simulink model "S"  (R2018b)
settings: Solver=ode14x  StartTime=0.0  StopTime=100  FixedStep=0.01  RelTol=1e-3
StopFcn:
  | figure;
  | plot(t,ref,'r--','linewidth',1.5);
  | hold on
  | plot(t,Ph,'k','linewidth',1.5);
  | legend('ref','Ph');
  | xlabel('events');ylabel('Ph(Mpa)');
  | grid on;
  | %%
  | figure
  | subplot(311)
  | plot(t,u,'k','linewidth',1);
  | ylabel('Voltage(v)');
  | hold on
  | legend('u')
  | grid on;
  | subplot(312)
  | plot(t,u_fbk,'k','linewidth',1.5);
  | ylabel('Voltage(v)');
  | legend('u_fbk');
  | hold on
  | grid on;
  | subplot(313)
  | plot(t,u_ffrk,'k','linewidth',1.5);
  | legend('u_ffrk');
  | xlabel('events');ylabel('Voltage(v)');
  | grid on;
  | %%
  | figure;
  | plot(t,rise,'k','linewidth',1.5);
  | hold on
  | plot(t,rise_r,'r--','linewidth',1.5);
  | legend('ref','Rising Duration');
  | xlabel('events');ylabel('Rising Duration(ms)');
  | grid on;
undefined symbols (not defined in the file or in its folder): sigbuilder_block
settings Model: Creator=sos h  LastModifiedBy=sistana
settings SolverCC: AlgebraicLoopSolver=LineSearch
settings SFSimCC: SimUseLocalCustomCode=off
settings RTWCC: RTWUseLocalCustomCode=off

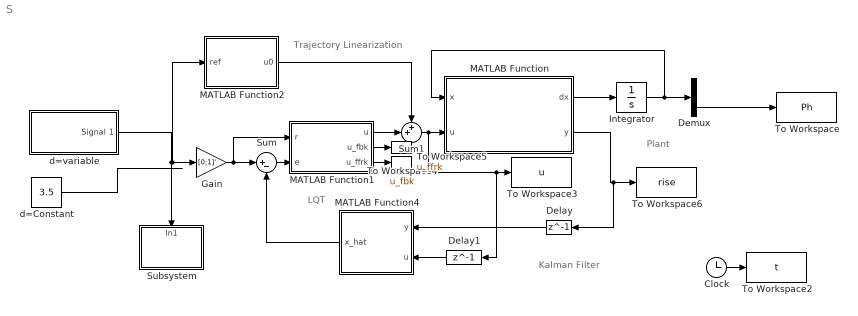
== system S ==
  note: Trajectory Linearization
  note: LQT
  note: Kalman Filter
  note: Plant
  Clock : Clock
  Delay : Delay  DelayLength=1
  Delay1 : Delay  DelayLength=1
  Demux : Demux  Outputs=2
  Gain : Gain  Gain=[0;1]'
  Integrator : Integrator  InitialCondition=[0.1;5]
  MATLAB Function : MATLAB Function  TreatAsAtomicUnit=on
  MATLAB Function1 : MATLAB Function  TreatAsAtomicUnit=on
  MATLAB Function2 : MATLAB Function  TreatAsAtomicUnit=on
  MATLAB Function4 : MATLAB Function  TreatAsAtomicUnit=on
  Subsystem : Subsystem
  Sum : Sum  Inputs=|+-
  Sum1 : Sum  Inputs=++|
  To Workspace : ToWorkspace  VariableName=Ph  SampleTime=-1
  To Workspace2 : ToWorkspace  VariableName=t  SampleTime=-1
  To Workspace3 : ToWorkspace  VariableName=u  SampleTime=-1
  To Workspace4 : ToWorkspace  VariableName=u_fbk  SampleTime=-1
  To Workspace5 : ToWorkspace  VariableName=u_ffrk  SampleTime=-1
  To Workspace6 : ToWorkspace  VariableName=rise  SampleTime=-1
  d=Constant : Constant  Value=3.5
  d=variable : Subsystem  Tag=STV Subsys  LoadFcn=sigbuilder_block('load');  StartFcn=sigbuilder_block('start');  StopFcn=sigbuilder_block('stop');  ClipboardFcn=sigbuilder_block('clipboard');  mask(Sigbuilder block){tuvar=[0:10]}
      mask help: Simulink:masks:SigbuilderBlock_MD
      mask init:
      | if ~strcmp(get_param(bdroot(gcbh),'SimulationStatus'),'stopped') tuvar = sigbuilder_block('maskInit'); end
      settings: CopyFcn=sigbuilder_block('copy');  DeleteFcn=sigbuilder_block('delete');  ModelCloseFcn=sigbuilder_block('modelClose');  PreSaveFcn=sigbuilder_block('preSave');  PauseFcn=sigbuilder_block('pause');  ContinueFcn=sigbuilder_block('continue');  NameChangeFcn=sigbuilder_block('namechange');  OpenFcn=sigbuilder_block('open',[437.25 153.75 550.5 359.25 ]);  CloseFcn=sigbuilder_block('close');
      mask Display: plot(0, 0, 100, 100,[2, 2, 32, 32, 2], [68, 8, 8, 68, 68],[32, 2], [38, 38], [32, 19, 2],[53, 60, 44], [32, 17, 17, 2],[16, 16, 31, 31]);txt = getActiveGroup(gcbh);text(2, 100, txt,'verticalAlignment', 'top');
  wires:
  MATLAB Function1/2(u_fbk) -> To Workspace4/1
  Integrator/1 -> Demux/1, MATLAB Function/1(x)
  Sum/1 -> MATLAB Function1/2(e)
  d=variable/1(Signal 1) -> Subsystem/1(In1), MATLAB Function2/1(ref), Gain/1
  MATLAB Function2/1(u0) -> Sum1/1
  Demux/2 -> To Workspace/1
  MATLAB Function1/3(u_ffrk) -> To Workspace5/1
  MATLAB Function1/1(u) -> Sum1/2
  MATLAB Function/1(dx) -> Integrator/1
  Gain/1 -> MATLAB Function1/1(r), Sum/1
  Sum1/1 -> Delay1/1, To Workspace3/1, MATLAB Function/2(u)
  MATLAB Function/2(y) -> Delay/1, To Workspace6/1
  Clock/1 -> To Workspace2/1
  MATLAB Function4/1(x_hat) -> Sum/2
  Delay/1 -> MATLAB Function4/1(y)
  Delay1/1 -> MATLAB Function4/2(u)
  d=Constant/1 -> ?

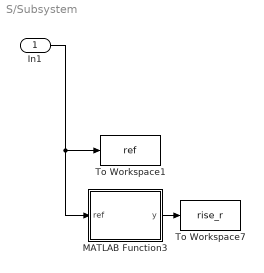
== system S/Subsystem ==
  In1 : Inport
  MATLAB Function3 : MATLAB Function  TreatAsAtomicUnit=on
  To Workspace1 : ToWorkspace  VariableName=ref  SampleTime=-1
  To Workspace7 : ToWorkspace  VariableName=rise_r  SampleTime=-1
  wires:
  In1/1 -> MATLAB Function3/1(ref), To Workspace1/1
  MATLAB Function3/1(y) -> To Workspace7/1

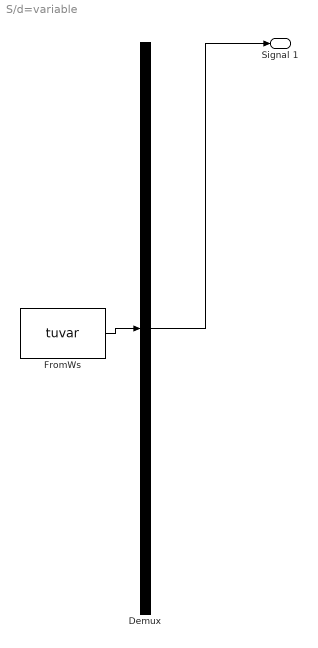
== system S/d=variable ==
  Demux : Demux  Tag=STV Demux  Outputs=1
  FromWs : FromWorkspace  Tag=STV FromWs  VariableName=tuvar  SampleTime=0
      SigBuilderData=|
      | common.afterFinalStr = 'Extrapolate'
      | common.sampleTime = 0
      | dataSet.timeRange = [0 200]
      | dataSet.name = 'Group 1'
      | sbobj.Groups.Name = 'Group 1'
      | sbobj.Groups.Signals.Name = 'Signal 1'
      | sbobj.Groups.Signals.XData = [0 25 25 50 75 75 120 120 166 166 200]
      | sbobj.Groups.Signals.YData = [7 7 9 9 9 7 7 9 9 7 7]
      | sbobj.Groups.TimeRange = [0 200]
  Signal 1 : Outport  Tag=STV Outport
  wires:
  Demux/1 -> Signal 1/1
  FromWs/1 -> Demux/1

== matlab function S/MATLAB Function1 ==
  settings: updateMethod=DISCRETE
  data: r input; e input; u output; u_fbk output; u_ffrk output
function [u,u_fbk,u_ffrk]  = fcn(r,e)
xk = r-e;
x = xk;
%% Parameters
k1 = -1.2*10^(-3);
k2 = 2.05;
tau1 = 0.38;
tau2 = 1;
c0 = -3.49;
a = 0.18;
b = -4.7;
c = 32.41;
Ts = 0.05;
%% 
Ak = [1-Ts/tau1 0
     (1/tau2-1/tau1)*Ts 1-Ts/tau2];
Bk = [0;Ts*k2/tau2];
Ck = [1 0
    0 2*a*x(2)+b];
persistent gk;
persistent Kk;
if (isempty(gk))
 F = 0.01*eye(2);
 gk = (Ck'*F*r);
 Kk = Ck'*F*Ck;
end
R = 1000;
Q = 1*[1 0;0 1];
%%
Lfbk = inv(R+Bk'*Kk*Bk)*Bk'*Kk*Ak;
Lffk = (inv(R+Bk'*Kk*Bk))'*Bk;   % 1*2
u_fbk = Lfbk*xk;
u_ffrk = Lffk'*gk;
for i =1:8
Kk = Ak'*Kk*inv([eye(2)-Bk*R^(-1)*Bk'*Kk])*Ak+Ck'*Q*Ck;
gk = Ak'*(eye(2)-Kk*inv(eye(2)+Bk*R^(-1)*Bk'*Kk)*Bk*inv(R)*Bk')*gk+Ck'*Q*r;

end
u = +u_fbk-u_ffrk;

== matlab function S/MATLAB Function ==
  settings: updateMethod=DISCRETE
  data: x input; dx output; u input; y output
function [dx,y] = fcn(x,u)
%% Parameters
k1 = -1.2*10^(-3);
k2 = 2.05;
tau1 = 0.38;
tau2 = 1;
c0 = -3.49;
a = 0.18;
b = -4.7;
c = 32.41;
Ts = 0.01;
%%
x=x+0.01*randn(1);
d = 1000;
dx = [-1/tau1*x(1)+k1/tau1*d;
      (1/tau2-1/tau1)*x(1)-1/tau2*x(2)+k2/tau2*u+k1/tau1*d];
y = a*x(2)^2+b*x(2)+c;

== matlab function S/MATLAB Function2 ==
  settings: updateMethod=DISCRETE
  data: u0 output; ref input
function u0 = fcn(ref)
u0=0;
if ref == 7
   u0 = 0.41*9.5935+0.0001*randn(1);%3.8537; %
end

if ref == 9
    
    u0 = 0.49*10.0542+0.0001*randn(1); %4.3143 ; 
end

== matlab function S/Subsystem/MATLAB Function3 ==
  settings: updateMethod=DISCRETE
  data: y output; ref input
function y = fcn(ref)
a = 0.18;
b = -4.7;
c = 32.41;
y = a*ref^2+b*ref+c;
end

== matlab function S/MATLAB Function4 ==
  settings: updateMethod=DISCRETE
  data: x_hat output; y input; u input
function x_hat = fcn(y,u)
k1 = -1.2*10^(-3);
k2 = 2.05;
tau1 = 0.38;
tau2 = 1;
c0 = -3.49;
a = 0.18;
b = -4.7;
c = 32.41;
Ts = 0.01;
%% 
Ak = [1-Ts/tau1 0
     (1/tau2-1/tau1)*Ts 1-Ts/tau2];
Bk = [0;Ts*k2/tau2];
Ck = [0 2*a*y+b];

persistent x
if(isempty(x))
 x = [0;0];   
end
Hk = 0.0011;
x = Ak*x+Bk*u+Hk*(y-Ck*x);
x_hat = x;

end
